simulink library "G_solar_function"  (R2025b)
settings: Solver=VariableStepAuto  StartTime=0.0  StopTime=10.0  RelTol=1e-3
settings Model: Creator=cdt  LastModifiedBy=cdt

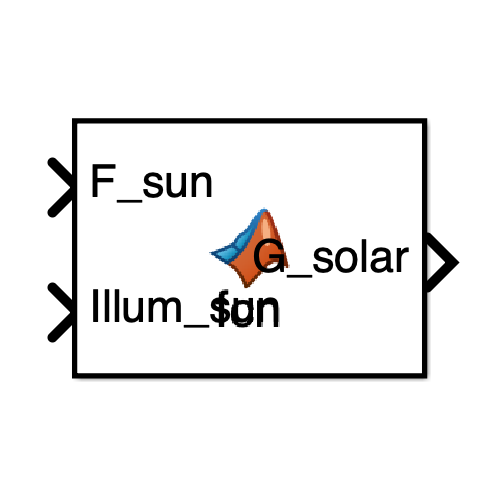
[thumbnail: Simulink's stored preview of the top-level diagram]
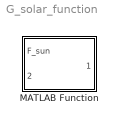
== system G_solar_function ==
  MATLAB Function : MATLAB Function  TreatAsAtomicUnit=on

== matlab function G_solar_function/MATLAB Function ==
  data: G_solar output; F_sun input; Illum_sun input
function G_solar = fcn(F_sun,Illum_sun)
%G_solar: total solbestråling på overfladen (W/m^2)
%alpha: sol-absorptans af materiale (forskellig for MLI og radiator)
%A: areal af overflade (m^2)
%F_sun: solens indfaldsvinkel-faktor (cos(theta) når solen rammer, 0 i skygge)
% Illum_sun: mellem 0 og 1, 0 = skygge, 1 = direkte sollys
G_s = 1361; % Solarkonstant W/m^2

G_solar = G_s * F_sun * Illum_sun;
